simulink model "stanley_1"  (R2025b)
settings: Solver=VariableStepAuto  StartTime=0.0  StopTime=10.0  RelTol=1e-3
settings Model: Creator=hubertm  LastModifiedBy=hubertm

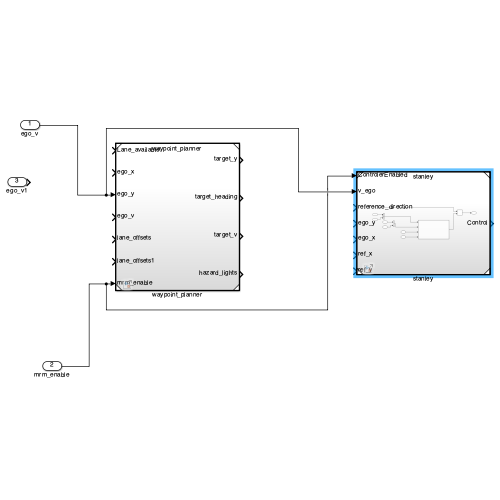
[thumbnail: Simulink's stored preview of the top-level diagram]
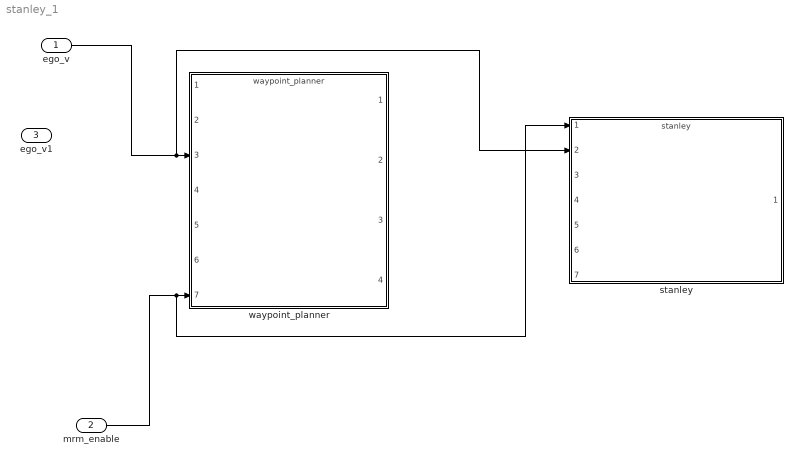
== system stanley_1 ==
  ego_v : Inport
  mrm_enable : Inport  Port=2
  ego_v1 : Inport  Port=3
  stanley : ModelReference  ModelNameDialog=stanley.slx  SimulationMode=Normal  ModelReferenceVersion=1.2
  waypoint_planner : ModelReference  ModelNameDialog=waypoint_planner.slx  SimulationMode=Normal  ModelReferenceVersion=1.4
  wires:
  ego_v/1 -> stanley/2, waypoint_planner/3
  mrm_enable/1 -> stanley/1, waypoint_planner/7
